simulink model "Model_NL"  (R2016b)
settings: Solver=VariableStepAuto  StartTime=0.0  StopTime=500  RelTol=1e-3
values from neighbouring files (symbols this model uses):
  dx = 2.86    [Parameters.m]
  dy = 32.5    [Parameters.m]
  dyaw = 0.26285    [Parameters.m]
  Iz = 1.10675    [Parameters.m]    (also in robustModel.m = Iz-0.22)
  l1 = 0.05    [Parameters.m]
  l2 = 0.05    [Parameters.m]
undefined symbols (not defined in the file or in its folder): F1, F2, F3, F4, l3, l4, mx, my
settings Model: Creator=USUARIO  LastModifiedBy=USUARIO
settings DataIOCC: Refine=100

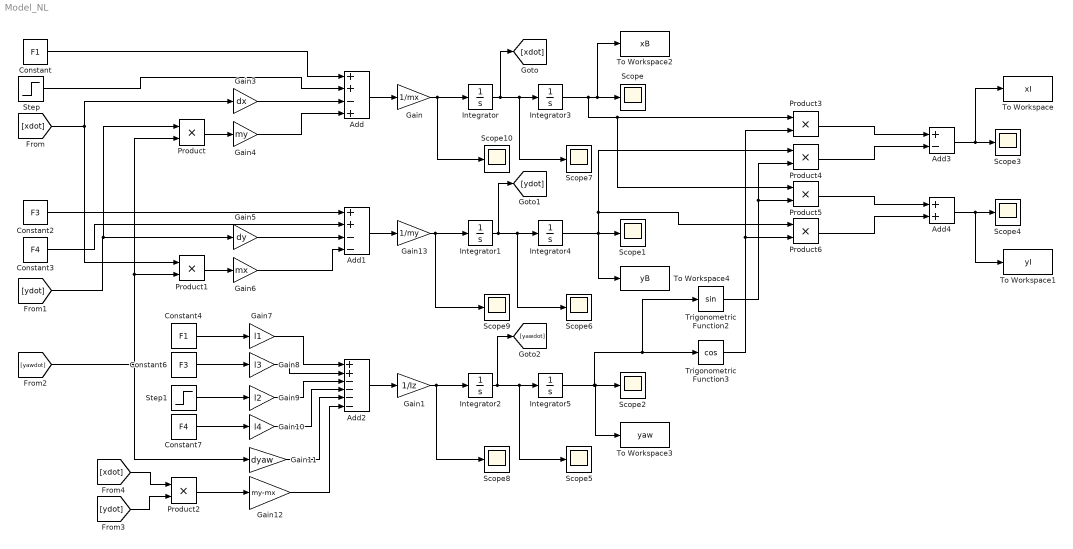
== system Model_NL ==
  Add : Sum  Inputs=++-+
  Add1 : Sum  Inputs=++--
  Add2 : Sum  Inputs=++----
  Add3 : Sum  Inputs=+-
  Add4 : Sum
  Constant : Constant  Value=F1
  Constant2 : Constant  Value=F3
  Constant3 : Constant  Value=F4
  Constant4 : Constant  Value=F1
  Constant6 : Constant  Value=F3
  Constant7 : Constant  Value=F4
  Gain : Gain  Gain=1/mx
  Gain1 : Gain  Gain=1/Iz
  Gain10 : Gain  Gain=l4
  Gain11 : Gain  Gain=dyaw
  Gain12 : Gain  Gain=my-mx
  Gain13 : Gain  Gain=1/my
  Gain3 : Gain  Gain=dx
  Gain4 : Gain  Gain=my
  Gain5 : Gain  Gain=dy
  Gain6 : Gain  Gain=mx
  Gain7 : Gain  Gain=l1
  Gain8 : Gain  Gain=l3
  Gain9 : Gain  Gain=l2
  Integrator{,1..5} (6 alike) : Integrator
  Product{,1..6} (7 alike) : Product
  Scope{,1..10} (11 alike) : Scope
  Step : Step  Time=100  Before=F2  After=0  SampleTime=0
  Step1 : Step  Time=100  Before=F2  After=0  SampleTime=0
  To Workspace : ToWorkspace  VariableName=xI  SaveFormat=Timeseries  SampleTime=-1
  To Workspace1 : ToWorkspace  VariableName=yI  SaveFormat=Timeseries  SampleTime=-1
  To Workspace2 : ToWorkspace  VariableName=xB  SaveFormat=Timeseries  SampleTime=-1
  To Workspace3 : ToWorkspace  VariableName=yaw  SaveFormat=Timeseries  SampleTime=-1
  To Workspace4 : ToWorkspace  VariableName=yB  SaveFormat=Timeseries  SampleTime=-1
  Trigonometric Function2 : Trigonometry
  Trigonometric Function3 : Trigonometry  Operator=cos
  wires:
  Add/1 -> Gain/1
  Add1/1 -> Gain13/1
  Add2/1 -> Gain1/1
  Integrator2/1 -> Scope5/1, Integrator5/1, [yawdot]
  Gain3/1 -> Add/3
  Gain4/1 -> Add/4
  Gain5/1 -> Add1/3
  Gain6/1 -> Add1/4
  Product/1 -> Gain4/1
  Product1/1 -> Gain6/1
  Gain7/1 -> Add2/1
  Gain8/1 -> Add2/2
  Gain9/1 -> Add2/3
  Gain10/1 -> Add2/4
  Gain11/1 -> Add2/5
  Gain12/1 -> Add2/6
  Constant/1 -> Add/1
  Step/1 -> Add/2
  Constant2/1 -> Add1/1
  Constant3/1 -> Add1/2
  [xdot] -> Product1/1, Gain3/1
  [ydot] -> Product/1, Gain5/1
  [yawdot] -> Gain11/1, Product1/2, Product/2
  Constant7/1 -> Gain10/1
  Step1/1 -> Gain9/1
  Constant6/1 -> Gain8/1
  Constant4/1 -> Gain7/1
  Product2/1 -> Gain12/1
  [ydot] -> Product2/2
  [xdot] -> Product2/1
  Integrator3/1 -> Product5/1, Product3/1, To Workspace2/1, Scope/1
  Integrator4/1 -> To Workspace4/1, Product6/1, Product4/1, Scope1/1
  Integrator5/1 -> To Workspace3/1, Scope2/1, Trigonometric Function2/1, Trigonometric Function3/1
  Trigonometric Function2/1 -> Product4/2, Product5/2
  Trigonometric Function3/1 -> Product3/2, Product6/2
  Product3/1 -> Add3/1
  Product4/1 -> Add3/2
  Product5/1 -> Add4/1
  Product6/1 -> Add4/2
  Add3/1 -> To Workspace/1, Scope3/1
  Add4/1 -> To Workspace1/1, Scope4/1
  Integrator1/1 -> Scope6/1, Integrator4/1, [ydot]
  Integrator/1 -> [xdot], Scope7/1, Integrator3/1
  Gain1/1 -> Scope8/1, Integrator2/1
  Gain13/1 -> Scope9/1, Integrator1/1
  Gain/1 -> Scope10/1, Integrator/1
